simulink model "soc_swhw_top"  (R2021a)
settings: Solver=VariableStepAuto  StartTime=0.0  StopTime=stopTime  RelTol=1e-3  EnableMultiTasking=on
InitFcn:
  | Initialize;
StartFcn:
  | Simulink.sdi.view;
StopFcn:
  | EvaluateOutput;
model workspace (MAT data in the model file):
  mmap = soc.memmap.MemoryMap
  mmap.isMapValid = 1
  mmap.controllerInfo = soc.memmap.MemController
  mmap.controllerInfo.baseAddr = '0x00000000'
  mmap.controllerInfo.size = '1024'
  mmap.controllerInfo.memConstraint = '0x40000000'
  mmap.controllerInfo.ipBaseAddr = 1073741824
  mmap.controllerInfo.ipAddrBridgeBase = 0
  mmap.map(1) = soc.memmap.MapParams
  mmap.map(1).area = 'Memory'
  mmap.map(1).name = 'Memory Channel'
  mmap.map(1).baseAddr = '0x00000000'
  mmap.map(1).size = '128'
  mmap.map(1).path = 'soc_swhw_top/Memory Channel'
  mmap.map(2) = soc.memmap.MapParams
  mmap.map(2).area = 'User Component'
  mmap.map(2).name = 'FPGA Algorithm Wrapper'
  mmap.map(2).baseAddr = '0x40010000'
  mmap.map(2).size = '64'
  mmap.map(2).path = 'soc_swhw_fpga/FPGA Algorithm Wrapper'
  mmap.map(2).regs(1) = soc.memmap.IPCoreRegParams
  mmap.map(2).regs(1).register = 'HDL Coder registers'
  mmap.map(2).regs(1).offset = '0x0000 - 0x00FF'
  mmap.map(2).regs(1).vectorlength = 'N/A'
  mmap.map(2).regs(1).type = 'Reserved'
  mmap.map(2).regs(1).reserved = 1
  mmap.map(2).regs(2) = soc.memmap.IPCoreRegParams
  mmap.map(2).regs(2).blkname = 'FPGA Algorithm Wrapper'
  mmap.map(2).regs(2).register = 'streamEnable'
  mmap.map(2).regs(2).offset = '0x0100'
  mmap.map(2).regs(2).vectorlength = '1'
  mmap.map(2).regs(2).type = 'Processor write channel'
  mmap.map(3) = soc.memmap.MapParams
  mmap.map(3).area = 'Implicit Component'
  mmap.map(3).name = 'DMARead'
  mmap.map(3).baseAddr = '0x40020000'
  mmap.map(3).size = '64'
  mwTaskManagerKernelLatency = 0
  socvcb = containers.Map
  socvcb.serialization.keys = {3.00024414062, 3.00036621094, 3.00048828125, 3.00085449219, 4.00024414062, 4.00036621094, 4.00048828125, 4.00085449219, 5.00024414062, 5.00036621094, 5.00048828125, 5.00085449219}
  socvcb.serialization.values : function handle (value not decoded)
  socvcb.serialization.uniformity = 0
  socvcb.serialization.keyType = 'double'
  socvcb.serialization.valueType = 'any'
values from neighbouring files (symbols this model uses):
  burstLen = 100    [Initialize.m]
  overlapWavIn = single(zeros((2 * length(inputWav) - frameSize),1))    [Initialize.m]
undefined symbols (not defined in the file or in its folder): AXI4, m, n, Stream
libraries: socmemlib x3, hwlogictestlib x2, proctasklib x1
PauseFcn:
  | EvaluateOutput;
settings Model: OrderedModelArguments=off  Creator=The MathWorks, Inc.  LastModifiedBy=AliReza
settings SolverCC: ConcurrentTasks=on  AlgebraicLoopSolver=TrustRegion  PositivePriorityOrder=on  AutoInsertRateTranBlk=on  InsertRTBMode=Never (minimum delay)
settings DataIOCC: ReturnWorkspaceOutputs=off
settings OptimizationCC: EnhancedBackFolding=on  PassReuseOutputArgsAs=Individual arguments  ZeroExternalMemoryAtStartup=off  ZeroInternalMemoryAtStartup=off  MaxStackSize=64  OptimizeBlockOrder=speed  DifferentSizesBufferReuse=on  OptimizationCustomize=off  EfficientTunableParamExpr=on
settings DebuggingCC: IntegerOverflowMsg=none  ParameterTunabilityLossMsg=error  SFMachineParentedDataDiag=warning  ArithmeticOperatorsInVariantConditions=warning
settings HardwareCC: ProdBitPerPointer=32  ProdBitPerSizeT=32  ProdBitPerPtrDiffT=32  ProdLargestAtomicInteger=Long  ProdLargestAtomicFloat=Double  ProdWordSize=32  ProdLongLongMode=on  ProdHWDeviceType=ARM Compatible->ARM Cortex  HardwareBoardFeatureSet=SoCBlockset
settings SFSimCC: SimUseLocalCustomCode=off  MATLABDynamicMemAlloc=off  CustomCodeUndefinedFunction=UseInterfaceOnly
settings RTWCC: SystemTargetFile=ert.tlc  HardwareBoard=Altera Cyclone V SoC development kit  TLCOptions="-aInlineSetEventsForThisBaseRateFcn=TLC_FALSE -aSuppressMultiTaskScheduler=TLC_FALSE  -aRateBasedStepFcn=0"  TemplateMakefile=ert_default_tmf  GenerateReport=on  RTWUseLocalCustomCode=off  Toolchain=ARM Development Studio Altera Edition (DS-5 AE)  LaunchReport=on
settings CodeAppCC: ForceParamTrailComments=on  IgnoreCustomStorageClasses=off  OperatorAnnotations=on  SimulinkDataObjDesc=on  SFDataObjDesc=on  InsertBlockDesc=on
settings ERTTargetCC: RootIOFormat=Structure reference

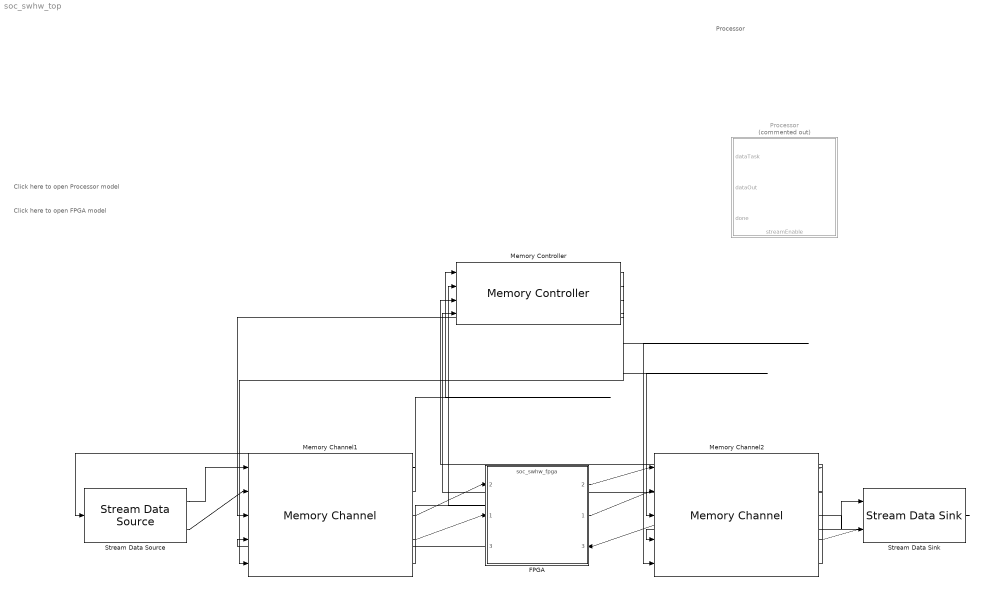
== system soc_swhw_top ==
  note: Click here to open FPGA model
  note: Processor
  note: Click here to open Processor model
  FPGA : ModelReference  ModelNameDialog=soc_swhw_fpga.slx  SimulationMode=Normal  ModelReferenceVersion=2.41
      settings: PortSchema="{\"entries\":[{\"content\":{\"sides\":[{\"content\":{\"connectorIds\":[\"Out2\",\"Out1\",\"In3\"]},\"type\":\"ConnectorPlacement.EquallySpacedRectSide\",\"uuid\":\"4ebd27d1-5bc0-4068-9441-99133dff9362\"},{\"content\":{\"connectorIds\":[\"In2\",\"In1\",\"Out3\"],\"side\":\"RIGHT\"},\"type\":\"ConnectorPlacement.EquallySpacedRectSide\",\"uuid\":\"18028c39-21e7-4f38-b500-7f7ea4fe36e5\"},{\"content\":{\"connectorIds\":[],\"side\":\"TOP\"},\"type\":\"ConnectorPlacement.EquallySpacedRectSide\",\"uuid\":\"457a3843-850c-4280-9c51-c37d0f6a5205\"},{\"content\":{\"connectorIds\":[],\"side\":\"BOTTOM\"},\"type\":\"ConnectorPlacement.EquallySpacedRectSide\",\"uuid\":\"47d097df-f43c-48ab-9e67-9c9a4b685d2e\"},{\"content\":{\"connectorIds\":[],\"side\":\"HIDDEN\"},\"type\":\"ConnectorPlacement.EquallySpacedRectSide\",\"uuid\":\"9dd4af0b-0c6a-42c5-bbd9-7d91ed33b034\"}]},\"type\":\"ConnectorPlacement.EquallySpacedConnector\",\"uuid\":\"2ce6b0d0-3283-4f33-a8e6-dc9a4f5a7eb7\"}],\"packageUris\":[\"http://schema.mathworks.com/mf0/Connector/R2020b\"],\"version\":\"1.0\"}"
  Memory Channel1 : socmemlib/Memory Channel  InstantiateOnLoad=on  ChannelType=AXI4-Stream FIFO  MRBufferSize=frameSize  MRNumBuffers=numBuffers  BurstLengthWriterChIf=burstLen  BurstLengthReaderChIf=burstLen  UseValuesFromTargetHardwareResources=on  ReaderWriterUseSameValues=on  FIFODepthWriter=8  FIFODepthReader=8  FIFOAFullDepthWriter=6  FIFOAFullDepthReader=6  ICClockFrequencyWriter=150  ICClockFrequencyReader=150  ICDataWidthWriter=64  ICDataWidthReader=64  ChDimensionsWriterChIf=1  ChTypeWriterChIf=single  ChFrameSampleTimeWriterChIf=sampleTime  ChBitPackedWriterChIf=off  OutSigSpecMatchesInSigSpec=on  ChDimensionsReaderChIf=1  ChTypeWithInhReaderChIf=uint32  ChFrameSampleTimeReaderChIf=1e-07  ChBitPackedReaderChIf=off  InsertInactivePixelClocksReaderChIf=off  FrameSizeReaderChIf=160x120p  ProtocolWriter=AXI4-Stream  ProtocolReader=AXI4-Stream  ChTypeReaderChIf=single  LastTargetBoard=Altera Cyclone V SoC development kit  Beta2Compatible=off  MRRegionSize=1600  DiagnosticLevel=No debug  MRBaseAddress=hex2dec('00010000')  UseTargetGlobalValues=off  InterruptHandlingTimeWriterChIf=10e-6  BufferEventIDWriterChIf=NOT_USED  BufferLengthReaderChIf=NOT_USED  InterruptHandlingTimeReaderChIf=10e-6  BufferEventIDReaderChIf=NOT_USED
      settings: SourceProductBaseCode=HW
  Memory Channel2 : socmemlib/Memory Channel  InstantiateOnLoad=on  ChannelType=AXI4-Stream FIFO  MRBufferSize=frameSize  MRNumBuffers=numBuffers  BurstLengthWriterChIf=burstLen  BurstLengthReaderChIf=burstLen  UseValuesFromTargetHardwareResources=on  ReaderWriterUseSameValues=on  FIFODepthWriter=8  FIFODepthReader=8  FIFOAFullDepthWriter=6  FIFOAFullDepthReader=6  ICClockFrequencyWriter=150  ICClockFrequencyReader=150  ICDataWidthWriter=64  ICDataWidthReader=64  ChDimensionsWriterChIf=1  ChTypeWriterChIf=single  ChFrameSampleTimeWriterChIf=sampleTime  ChBitPackedWriterChIf=off  OutSigSpecMatchesInSigSpec=on  ChDimensionsReaderChIf=1  ChTypeWithInhReaderChIf=uint32  ChFrameSampleTimeReaderChIf=1e-07  ChBitPackedReaderChIf=off  InsertInactivePixelClocksReaderChIf=off  FrameSizeReaderChIf=160x120p  ProtocolWriter=AXI4-Stream  ProtocolReader=AXI4-Stream  ChTypeReaderChIf=single  LastTargetBoard=Altera Cyclone V SoC development kit  Beta2Compatible=off  MRRegionSize=1600  DiagnosticLevel=No debug  MRBaseAddress=hex2dec('00010000')  UseTargetGlobalValues=off  InterruptHandlingTimeWriterChIf=10e-6  BufferEventIDWriterChIf=NOT_USED  BufferLengthReaderChIf=NOT_USED  InterruptHandlingTimeReaderChIf=10e-6  BufferEventIDReaderChIf=NOT_USED
      settings: SourceProductBaseCode=HW
  Memory Controller : socmemlib/Memory Controller  InstantiateOnLoad=on  NumMasters=4  ICArbitrationPolicy=Round robin  UseValuesFromTargetHardwareResources=on  ControllerFrequency=150  ControllerDataWidth=64  BandwidthDerating=2.3  WriteFirstTransferLatency=4  ReadFirstTransferLatency=5  WriteLastTransferLatency=4  ReadLastTransferLatency=1  LastTargetBoard=Altera Cyclone V SoC development kit  DiagnosticLevel=No debug  MAX_NUM_MASTERS=12  DDRRefreshLength=4  DDRRefreshInterval=7.8  PlotTimeResolution=3000*60e-7
      settings: SourceProductBaseCode=HW
  Processor : Subsystem  Commented=on
      settings: PortSchema="{\"entries\":[{\"content\":{\"sides\":[{\"content\":{\"connectorIds\":[\"In1\",\"Out2\",\"In2\"]},\"type\":\"ConnectorPlacement.EquallySpacedRectSide\",\"uuid\":\"907b3a56-763a-42ee-85ff-5e1ce14deb7d\"},{\"content\":{\"connectorIds\":[],\"side\":\"RIGHT\"},\"type\":\"ConnectorPlacement.EquallySpacedRectSide\",\"uuid\":\"ad6a187b-3ae8-4811-8877-d9e2be6fa16c\"},{\"content\":{\"connectorIds\":[],\"side\":\"TOP\"},\"type\":\"ConnectorPlacement.EquallySpacedRectSide\",\"uuid\":\"6e54ea57-de3c-42ee-94cd-fde1030cf300\"},{\"content\":{\"connectorIds\":[\"Out1\"],\"side\":\"BOTTOM\"},\"type\":\"ConnectorPlacement.EquallySpacedRectSide\",\"uuid\":\"1350198a-8208-4c6e-8d71-6a3dfa7e18c3\"},{\"content\":{\"connectorIds\":[],\"side\":\"HIDDEN\"},\"type\":\"ConnectorPlacement.EquallySpacedRectSide\",\"uuid\":\"bc18f407-0946-4df8-8419-3e94766db50a\"}]},\"type\":\"ConnectorPlacement.EquallySpacedConnector\",\"uuid\":\"65011cd7-483b-4b9d-803c-3fa4b2312ee3\"}],\"packageUris\":[\"http://schema.mathworks.com/mf0/Connector/R2020b\"],\"version\":\"1.0\"}"
  Stream Data Sink : hwlogictestlib/Stream Data Sink  SaveData=on  SavedName=overlapWavOut
      settings: SourceProductBaseCode=HW
  Stream Data Source : hwlogictestlib/Stream Data Source  ChType=single  ChDimensions=1  BufferLen=burstLen  TotalTransfers=floor(length(overlapWavIn)/burstLen)  DataGenMode=workspace  CntrInitValue=0  VbleName=overlapWavIn  DataVbleName="\"overlapWavIn\""  ChFrameSampleTime=sampleTime  InitDelay=0  RandomDelayIT=off  minDelay=3  maxDelay=6  trnsfrdelay=0  ErraticMode=off  EMProb=1  ChWidth=32  ChLength=1  ChCompLength=1  ChContainerType=single  ChTLASTCount=100  CHFLATTENLEN=1
      settings: SourceProductBaseCode=HW
  wires:
  Memory Controller/2 -> Memory Channel1/5
  Memory Channel1/5 -> Memory Controller/2
  Memory Controller/1 -> Memory Channel1/3
  Memory Channel1/2 -> Memory Controller/1
  Stream Data Source/1 -> Memory Channel1/1
  Stream Data Source/2 -> Memory Channel1/2
  Memory Channel1/1 -> Stream Data Source/1
  Memory Channel1/3 -> FPGA/2
  Memory Channel1/4 -> FPGA/1
  FPGA/1 -> Memory Channel2/2
  Stream Data Sink/1 -> Memory Channel2/4
  Memory Channel2/4 -> Stream Data Sink/2
  Memory Channel2/3 -> Stream Data Sink/1
  FPGA/2 -> Memory Channel2/1
  FPGA/3 -> Memory Channel1/4
  Memory Channel2/1 -> FPGA/3
  Memory Controller/4 -> Memory Channel2/5
  Memory Channel2/5 -> Memory Controller/4
  Memory Channel2/2 -> Memory Controller/3
  Memory Controller/3 -> Memory Channel2/3

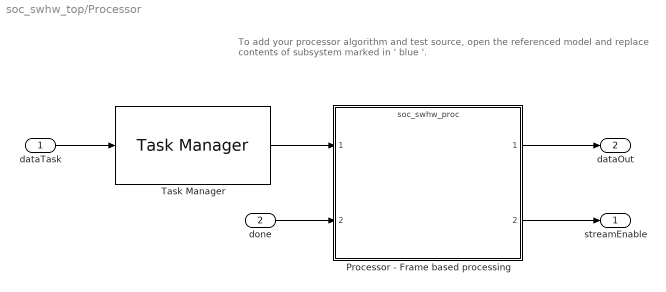
== system soc_swhw_top/Processor ==
  note: To add your processor algorithm and test source, open the referenced
      | model and replace contents of subsystem marked in ' blue '.
  dataTask : Inport
  done : Inport  Port=2
  Processor - Frame based processing : ModelReference  InputPortMessageModes=n,m  OutputPortMessageModes=m,m  ModelNameDialog=soc_swhw_proc.slx  SimulationMode=Normal  ModelReferenceVersion=2.0
  Task Manager : proctasklib/Task Manager  AllTaskData="{\"taskName\":\"dataWriteTask\",\"taskType\":\"Event-driven\",\"taskEvent\":\"dataWriteTaskEvent\",\"taskPeriod\":\"0.018\",\"taskPriority\":\"50\",\"coreSelection\":\"Specified core\",\"coreNum\":\"0\",\"dropOverranTasks\":false,\"playbackRecorded\":false,\"diagnosticsFile\":\"Z:\\\\24\\\\athakkar.May7\\\\work\\\\Vivado_prj\\\\soc_getting_started_top_sw_diagnostics\\\\hw\\\\2018_5_18_17_17_55\\\\dataReadTask.csv\",\"taskDurationSource\":\"Dialog\",\"taskDuration\":0.003,\"taskDurationDeviation\":0,\"logExecutionData\":true,\"logDroppedTasks\":false,\"version\":\"2.2\",\"taskDurationData\":{\"percent\":[\"100\"],\"mean\":[\"0.35e-3\"],\"dev\":[\"0\"],\"min\":[\"0.35e-3\"],\"max\":[\"0.35e-3\"]},\"taskEventSource\":\"Unspecified\"}"  EnableTaskSimulation=on  StreamToSDI=on  WriteToFile=off  OverwriteFile=off  SupportEventPorts=on
      settings: SourceProductBaseCode=HW
  streamEnable : Outport
  dataOut : Outport  Port=2  VectorParamsAs1DForOutWhenUnconnected=off
  wires:
  done/1 -> Processor - Frame based processing/2
  Processor - Frame based processing/1 -> dataOut/1
  dataTask/1 -> Task Manager/1
  Task Manager/1 -> Processor - Frame based processing/1
  Processor - Frame based processing/2 -> streamEnable/1
